simulink model "msd_resonant_frequency_seeking_CT"  (R2024b)
settings: Solver=ode4  StartTime=0.0  StopTime=Tfin  FixedStep=Ts  RelTol=1e-3
values from neighbouring files (symbols this model uses):
  A_cmd = 1    [msd_resonant_frequency_seeking_CT_run.m]    (also in msd_resonant_frequency_seeking_DT_run.m; msd_resonant_frequency_seeking_DT_vanishing_dither_run.m)
  A_esc_d = 1    [msd_resonant_frequency_seeking_CT_run.m]    (also in msd_resonant_frequency_seeking_DT_run.m = 1.2; msd_resonant_frequency_seeking_DT_vanishing_dither_run.m = 1.2)
  A_esc_m = 1    [msd_resonant_frequency_seeking_CT_run.m]    (also in msd_resonant_frequency_seeking_DT_run.m = 1.2)
  c = 2    [msd_frequency_response_magnitude.m]    (also in msd_resonant_frequency_seeking_CT_run.m; msd_resonant_frequency_seeking_DT_run.m; msd_resonant_frequency_seeking_DT_vanishing_dither_run.m)
  k = 1000    [msd_frequency_response_magnitude.m]    (also in msd_resonant_frequency_seeking_CT_run.m; msd_resonant_frequency_seeking_DT_run.m; msd_resonant_frequency_seeking_DT_vanishing_dither_run.m)
  K_esc = 2.5    [msd_resonant_frequency_seeking_CT_run.m]    (also in msd_resonant_frequency_seeking_DT_run.m = 2; msd_resonant_frequency_seeking_DT_vanishing_dither_run.m)
  K_g = 500    [msd_resonant_frequency_seeking_CT_run.m]    (also in msd_resonant_frequency_seeking_DT_run.m; msd_resonant_frequency_seeking_DT_vanishing_dither_run.m)
  lambda_osc = 1    [msd_resonant_frequency_seeking_CT_run.m]    (also in msd_resonant_frequency_seeking_DT_run.m; msd_resonant_frequency_seeking_DT_vanishing_dither_run.m)
  m = 1    [msd_frequency_response_magnitude.m]    (also in msd_resonant_frequency_seeking_CT_run.m; msd_resonant_frequency_seeking_DT_run.m; msd_resonant_frequency_seeking_DT_vanishing_dither_run.m)
  omega_cmd_0 = 20    [msd_resonant_frequency_seeking_CT_run.m]    (also in msd_resonant_frequency_seeking_DT_run.m; msd_resonant_frequency_seeking_DT_vanishing_dither_run.m)
  omega_esc = 1    [msd_resonant_frequency_seeking_CT_run.m]    (also in msd_resonant_frequency_seeking_DT_run.m; msd_resonant_frequency_seeking_DT_vanishing_dither_run.m = 4)
  omega_h = 2    [msd_resonant_frequency_seeking_CT_run.m]    (also in msd_resonant_frequency_seeking_DT_run.m = 0.1; msd_resonant_frequency_seeking_DT_vanishing_dither_run.m = 3)
  omega_l = 4    [msd_resonant_frequency_seeking_CT_run.m]    (also in msd_resonant_frequency_seeking_DT_run.m; msd_resonant_frequency_seeking_DT_vanishing_dither_run.m = 10)
  T_d = 2    [msd_resonant_frequency_seeking_CT_run.m]
  t_stop = 300    [msd_resonant_frequency_seeking_CT_run.m]    (also in msd_resonant_frequency_seeking_DT_run.m)
  x0 = [0;0]    [msd_resonant_frequency_seeking_CT_run.m]    (also in msd_resonant_frequency_seeking_DT_run.m; msd_resonant_frequency_seeking_DT_vanishing_dither_run.m; nonlinear_oscillator_frequency_switch_test.m = [0.0; 1.0])
settings Model: Creator=Juan Augusto Paredes  LastModifiedBy=Juan Augusto Paredes
settings RTWCC: GPUComputeCapability=3.5

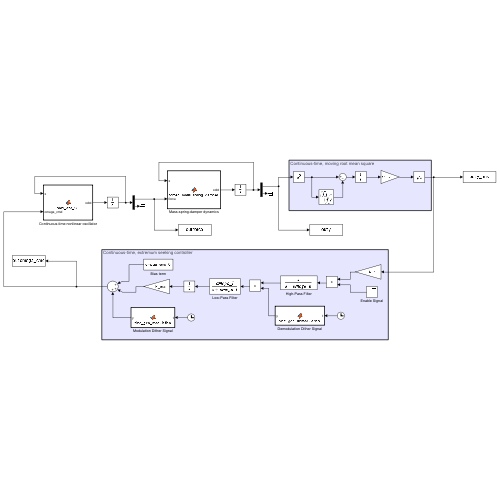
[thumbnail: Simulink's stored preview of the top-level diagram]
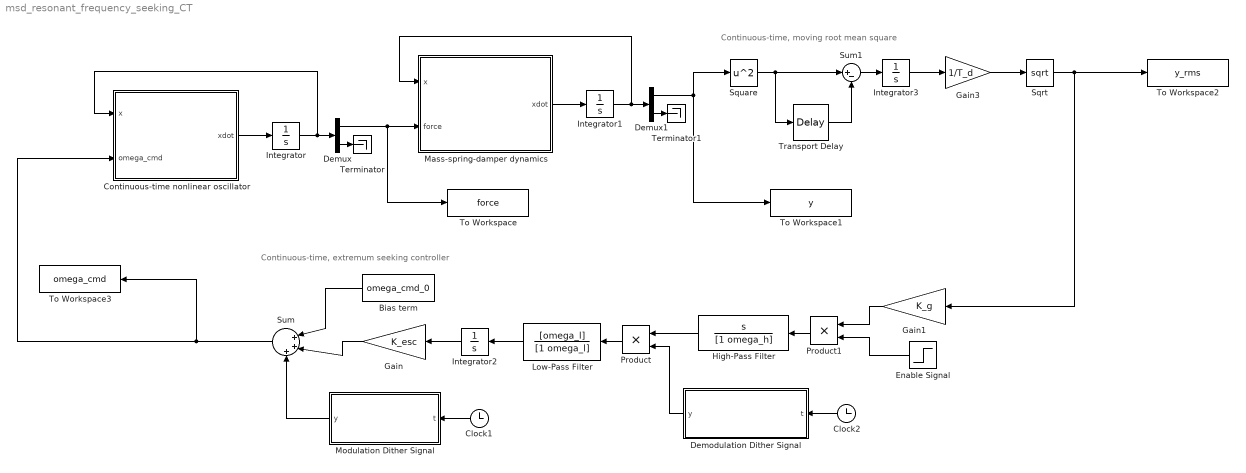
== system msd_resonant_frequency_seeking_CT ==
  note: Continuous-time, extremum seeking controller
  note: Continuous-time, moving root mean square
  Bias term : Constant  Value=omega_cmd_0
  Clock1 : Clock
  Clock2 : Clock
  Continuous-time nonlinear oscillator : MATLAB Function  TreatAsAtomicUnit=on
  Demodulation Dither Signal : MATLAB Function  TreatAsAtomicUnit=on
  Demux : Demux  Outputs=2
  Demux1 : Demux  Outputs=2
  Enable Signal : Step  Time=2*T_d  SampleTime=0
  Gain : Gain  Gain=K_esc
  Gain1 : Gain  Gain=K_g
  Gain3 : Gain  Gain=1/T_d
  High-Pass Filter : TransferFcn  Numerator=[1 0]  Denominator=[1 omega_h]
  Integrator : Integrator  InitialCondition="[0;  A_cmd]"
  Integrator1 : Integrator  InitialCondition=x0
  Integrator2 : Integrator
  Integrator3 : Integrator
  Low-Pass Filter : TransferFcn  Numerator=[omega_l]  Denominator=[1 omega_l]
  Mass-spring-damper dynamics : MATLAB Function  TreatAsAtomicUnit=on
  Modulation Dither Signal : MATLAB Function  TreatAsAtomicUnit=on
  Product : Product
  Product1 : Product
  Sqrt : Sqrt
  Square : Math  Operator=square
  Sum : Sum  Inputs=|+++
  Sum1 : Sum  Inputs=|+-
  Terminator : Terminator
  Terminator1 : Terminator
  To Workspace : ToWorkspace  VariableName=force  SampleTime=-1
  To Workspace1 : ToWorkspace  VariableName=y  SampleTime=-1
  To Workspace2 : ToWorkspace  VariableName=y_rms  SampleTime=-1
  To Workspace3 : ToWorkspace  VariableName=omega_cmd  SampleTime=-1
  Transport Delay : TransportDelay  DelayTime=T_d  BufferSize=3072
  wires:
  Continuous-time nonlinear oscillator/1(xdot) -> Integrator/1
  Integrator/1 -> Demux/1, Continuous-time nonlinear oscillator/1(x)
  Demux/2 -> Terminator/1
  Demux/1 -> To Workspace/1, Mass-spring-damper dynamics/2(force)
  Mass-spring-damper dynamics/1(xdot) -> Integrator1/1
  Integrator1/1 -> Demux1/1, Mass-spring-damper dynamics/1(x)
  Demux1/2 -> Terminator1/1
  Transport Delay/1 -> Sum1/2
  Gain3/1 -> Sqrt/1
  Square/1 -> Sum1/1, Transport Delay/1
  Demux1/1 -> Square/1, To Workspace1/1
  Sum1/1 -> Integrator3/1
  Integrator3/1 -> Gain3/1
  Sum/1 -> To Workspace3/1, Continuous-time nonlinear oscillator/2(omega_cmd)
  Sqrt/1 -> Gain1/1, To Workspace2/1
  Modulation Dither Signal/1(y) -> Sum/3
  Gain/1 -> Sum/2
  Bias term/1 -> Sum/1
  Gain1/1 -> Product1/1
  Enable Signal/1 -> Product1/2
  Demodulation Dither Signal/1(y) -> Product/2
  Product/1 -> Low-Pass Filter/1
  Integrator2/1 -> Gain/1
  High-Pass Filter/1 -> Product/1
  Clock2/1 -> Demodulation Dither Signal/1(t)
  Clock1/1 -> Modulation Dither Signal/1(t)
  Product1/1 -> High-Pass Filter/1
  Low-Pass Filter/1 -> Integrator2/1

== matlab function msd_resonant_frequency_seeking_CT/Mass-spring-damper dynamics ==
  settings: updateMethod=CONTINUOUS
  data: x input size=2; xdot output size=2; force input size=1; m parameter size=1; k parameter size=1; c parameter size=1
function xdot = forced_mass_spring_damper(x,force, m, k, c)
    xdot = [0 1; -k/m -c/m]*x + [0;1/m]*force;
end

== matlab function msd_resonant_frequency_seeking_CT/Continuous-time nonlinear oscillator ==
  settings: updateMethod=CONTINUOUS
  data: x input size=2; xdot output size=2; omega_cmd input size=1; A_cmd parameter size=1; lambda_osc parameter size=1
function xdot = nonl_osc_CT(x, omega_cmd, A_cmd, lambda_osc)
    % Continuous-time, nonlinear oscillator dynamics
    xdot = ([0 omega_cmd; -omega_cmd 0] - lambda_osc*((x.'*x)- A_cmd^2)*eye(2))*x;

end

== matlab function msd_resonant_frequency_seeking_CT/Modulation Dither Signal ==
  data: t input size=1; y output size=1; A_esc_m parameter size=1; omega_esc parameter size=1; t_stop parameter size=1
function y = sine_gen_modulation(t, A_esc_m, omega_esc, t_stop)

    y = A_esc_m*sin(omega_esc*t);
    if t > t_stop
        y = 0;
    end

end

== matlab function msd_resonant_frequency_seeking_CT/Demodulation Dither Signal ==
  data: t input size=1; y output size=1; A_esc_d parameter size=1; omega_esc parameter size=1
function y = sine_gen_demodulation(t, A_esc_d, omega_esc)

    y = A_esc_d*sin(omega_esc*t);

end
